simulink model "Rocket_Simulation"  (R2024a)
settings: Solver=VariableStepAuto  StartTime=0.0  StopTime=25  RelTol=1e-3
values from neighbouring files (symbols this model uses):
  g = -9.80665    [OpenRocketDataLoader.m]
undefined symbols (not defined in the file or in its folder): magnitude
libraries: simulink x6, aerolibactuator x1, aerolibatmos2 x1
settings Model: Creator=bennettbabu  LastModifiedBy=mason

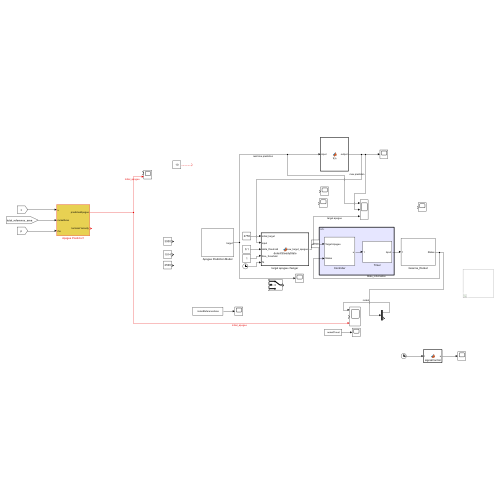
[thumbnail: Simulink's stored preview of the top-level diagram]
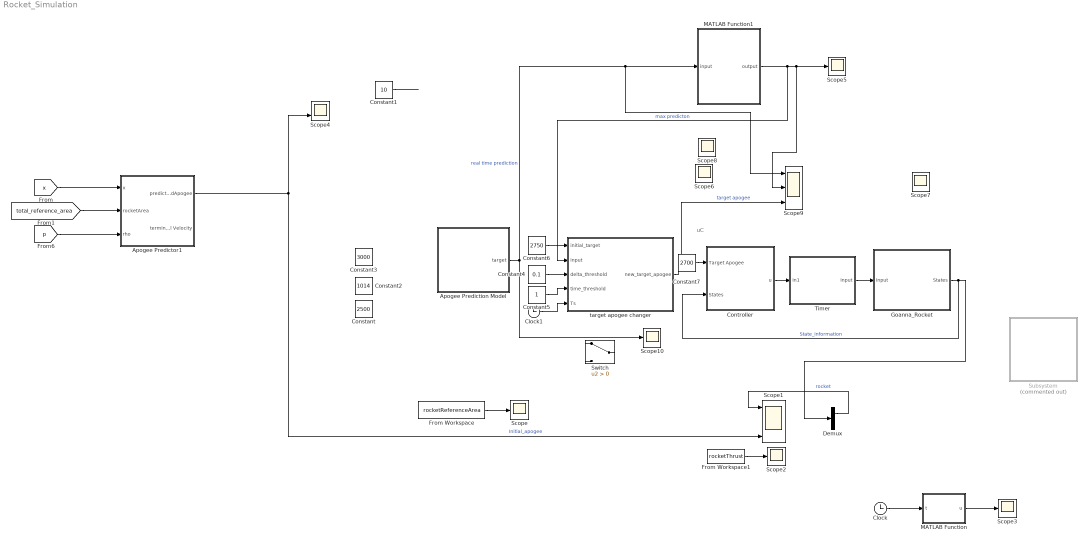
== system Rocket_Simulation ==
  note: uC
  Apogee Prediction Model : Subsystem
  Apogee Predictor1 : Subsystem
  Clock : Clock
  Clock1 : Clock
  Constant : Constant  Value=2500
  Constant1 : Constant  Value=10
  Constant2 : Constant  Value=1014
  Constant3 : Constant  Value=3000
  Constant4 : Constant  Value=0.1
  Constant5 : Constant
  Constant6 : Constant  Value=2750
  Constant7 : Constant  Value=2700
  Controller : Subsystem
  Demux : Demux  Outputs=2
  From Workspace : FromWorkspace  VariableName=rocketReferenceArea
  From Workspace1 : FromWorkspace  VariableName=rocketThrust
  Goanna_Rocket : Subsystem
  MATLAB Function : MATLAB Function  TreatAsAtomicUnit=on
  MATLAB Function1 : MATLAB Function  TreatAsAtomicUnit=on  SystemSampleTime=0.01
  Scope{,2..3,5..8,10} (8 alike) : Scope
  Scope1 : Scope  NumInputPorts=3
  Scope4 : Scope  NumInputPorts=2
  Scope9 : Scope  NumInputPorts=3
  Subsystem : Subsystem  Commented=on
  Switch : Switch  Criteria=u2 > Threshold  SaturateOnIntegerOverflow=off  InputSameDT=off
  Timer : Subsystem
  target apogee changer : MATLAB Function  TreatAsAtomicUnit=on  SystemSampleTime=0.01
  wires:
  Goanna_Rocket/1(States) -> Demux/1, Controller/2(States)  "State_information"
  Controller/1(u) -> Timer/1(In1)
  From Workspace/1 -> Scope/1
  Demux/1 -> Scope1/1  "rocket"
  From Workspace1/1 -> Scope2/1
  Clock/1 -> MATLAB Function/1(t)
  MATLAB Function/1(u) -> Scope3/1
  [p] -> Apogee Predictor1/3(rho)
  [total_reference_area] -> Apogee Predictor1/2(rocketArea)
  [x] -> Apogee Predictor1/1(x)
  MATLAB Function1/1(output) -> target apogee changer/2(input), Scope9/2, Scope5/1  "max predicton"
  Apogee Predictor1/1(predictedApogee) -> Scope1/3, Scope4/2  "Initial_apogee"
  Constant1/1 -> ?
  target apogee changer/1(new_target_apogee) -> Scope9/3  "target apogee"
  Constant4/1 -> target apogee changer/3(delta_threshold)
  Constant5/1 -> target apogee changer/4(time_threshold)
  Clock1/1 -> target apogee changer/5(Ts)
  Apogee Prediction Model/1(target) -> Scope9/1, MATLAB Function1/1(input), Scope10/1  "real time prediction"
  Constant6/1 -> target apogee changer/1(initial_target)
  Constant7/1 -> Controller/1(Target Apogee)
  Timer/1(Input) -> Goanna_Rocket/1(Input)

== system Rocket_Simulation/Apogee Prediction Model ==
  Idealised Curve (Covers the middle Cd and Airbrake Area) : Subsystem
  Multiply : Gain  Gain=1.0
  Scope : Scope
  Terminator : Terminator
  target : Outport
  wires:
  [p] -> Idealised Curve (Covers the middle Cd and Airbrake Area)/2(rho)
  [x] -> Idealised Curve (Covers the middle Cd and Airbrake Area)/1(x)
  Idealised Curve (Covers the middle Cd and Airbrake Area)/1(predictedApogee) -> Multiply/1  "Initial_apogee"
  Multiply/1 -> Scope/1, target/1  "target"
  Idealised Curve (Covers the middle Cd and Airbrake Area)/2(terminal Velocity) -> Terminator/1

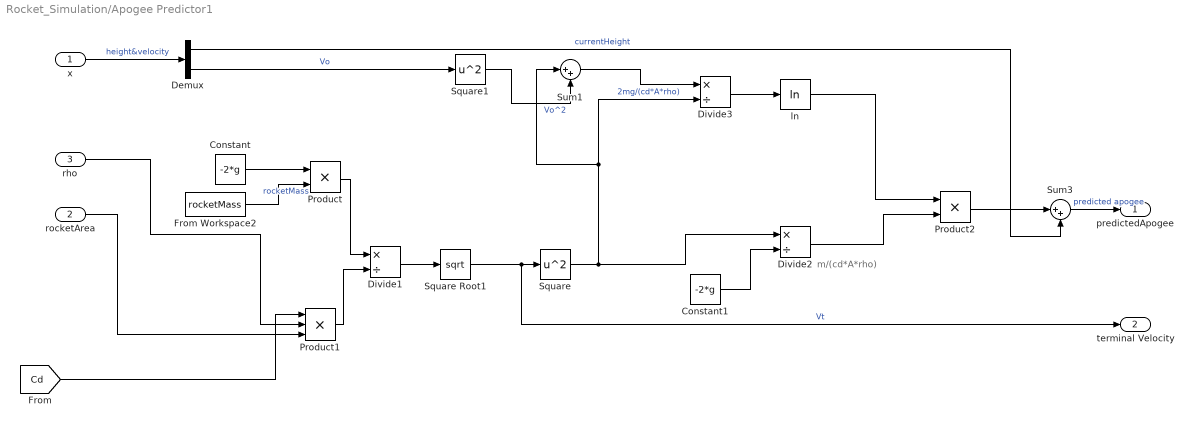
== system Rocket_Simulation/Apogee Predictor1 ==
  note: m/(cd*A*rho)
  x : Inport
  rocketArea : Inport  Port=2
  rho : Inport  Port=3
  Constant : Constant  Value=-2*g
  Constant1 : Constant  Value=-2*g
  Demux : Demux  Outputs=2
  Divide1 : Product  Inputs=*/
  Divide2 : Product  Inputs=*/
  Divide3 : Product  Inputs=*/
  From Workspace2 : FromWorkspace  VariableName=rocketMass
  Product : Product
  Product1 : Product  Inputs=3
  Product2 : Product
  Square : Math  Operator=square
  Square Root1 : Sqrt
  Square1 : Math  Operator=square
  Sum1 : Sum  Inputs=|++
  Sum3 : Sum  Inputs=|++
  ln : Math  Operator=log
  predictedApogee : Outport
  terminal Velocity : Outport  Port=2
  wires:
  Constant/1 -> Product/1
  Product/1 -> Divide1/1
  Product1/1 -> Divide1/2
  [Cd] -> Product1/1
  rho/1 -> Product1/2
  rocketArea/1 -> Product1/3
  Divide1/1 -> Square Root1/1
  Square Root1/1 -> terminal Velocity/1, Square/1  "Vt"
  Product2/1 -> Sum3/1
  ln/1 -> Product2/1
  Divide2/1 -> Product2/2
  Square/1 -> Divide3/2, Sum1/1, Divide2/1  "2mg/(cd*A*rho)"
  Constant1/1 -> Divide2/2
  Divide3/1 -> ln/1
  Square1/1 -> Sum1/2  "Vo^2"
  Sum1/1 -> Divide3/1
  x/1 -> Demux/1  "height&velocity"
  From Workspace2/1 -> Product/2  "rocketMass"
  Demux/2 -> Square1/1  "Vo"
  Demux/1 -> Sum3/2  "currentHeight"
  Sum3/1 -> predictedApogee/1  "predicted apogee"

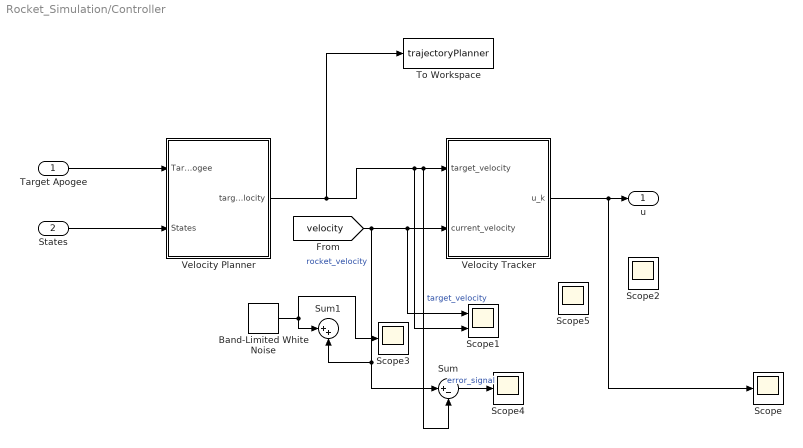
== system Rocket_Simulation/Controller ==
  Target Apogee : Inport
  States : Inport  Port=2
  Band-Limited White Noise : simulink/Sources/Band-Limited White Noise  Cov=[0.00001]  Ts=0.001  seed=[23341]
  Scope{,2..5} (5 alike) : Scope
  Scope1 : Scope  NumInputPorts=2
  Sum : Sum  Inputs=|+-
  Sum1 : Sum  Inputs=|++
  To Workspace : ToWorkspace  VariableName=trajectoryPlanner  SaveFormat=Timeseries  SampleTime=-1
  Velocity Planner : Subsystem
  Velocity Tracker : Subsystem
  u : Outport
  wires:
  Target Apogee/1 -> Velocity Planner/1(Target Apogee)
  States/1 -> Velocity Planner/2(States)
  Velocity Tracker/1(u_k) -> Scope/1, u/1
  [velocity] -> Sum1/2, Sum/1, Velocity Tracker/2(current_velocity), Scope1/1  "rocket_velocity"
  Velocity Planner/1(target_velocity) -> To Workspace/1, Sum/2, Velocity Tracker/1(target_velocity), Scope1/2  "target_velocity"
  Band-Limited White Noise/1 -> Scope3/1, Sum1/1
  Sum/1 -> Scope4/1  "error_signal"

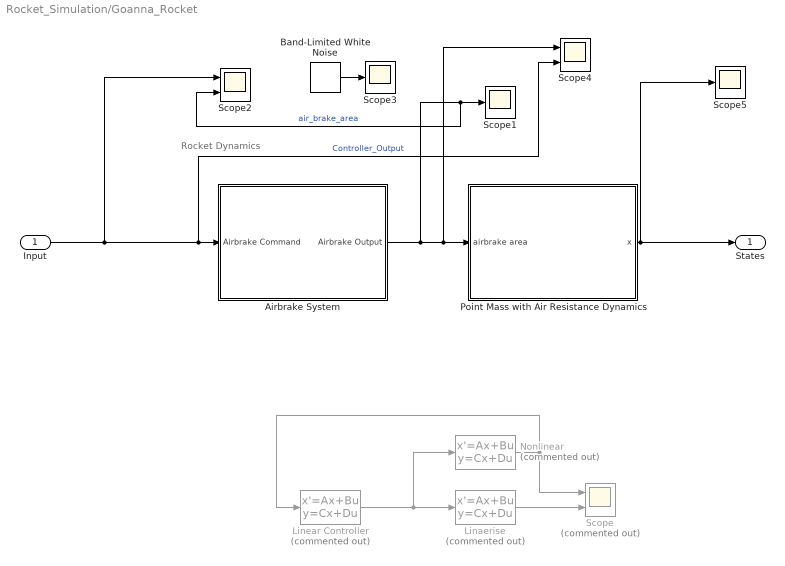
== system Rocket_Simulation/Goanna_Rocket ==
  note: Rocket Dynamics
  Input : Inport
  Airbrake System : Subsystem
      mask Display: image('airbrake.png');
  Band-Limited White Noise : simulink/Sources/Band-Limited White Noise  Cov=[0.0001]  Ts=0.1  seed=[23341]
  "Linaerise " : StateSpace  Commented=on  InitialCondition=0
  Linear Controller : StateSpace  Commented=on  InitialCondition=0
  Nonlinear : StateSpace  Commented=on  InitialCondition=0
  "Point Mass with Air Resistance Dynamics " : Subsystem
      mask Display: image('rocket.jpeg');
  Scope : Scope  Commented=on  NumInputPorts=2
  Scope1 : Scope
  Scope2 : Scope  NumInputPorts=2
  Scope3 : Scope
  Scope4 : Scope  NumInputPorts=2
  Scope5 : Scope
  States : Outport
  wires:
  Linear Controller/1 -> Nonlinear/1, "Linaerise "/1
  Nonlinear/1 -> Linear Controller/1, Scope/1
  "Linaerise "/1 -> Scope/2
  Input/1 -> Scope2/1, Scope4/2, Airbrake System/1(Airbrake Command)  "Controller_Output"
  Airbrake System/1(Airbrake Output) -> Scope4/1, "Point Mass with Air Resistance Dynamics "/1(airbrake area), Scope2/2, Scope1/1  "air_brake_area"
  Band-Limited White Noise/1 -> Scope3/1
  "Point Mass with Air Resistance Dynamics "/1(x) -> Scope5/1, States/1

== system Rocket_Simulation/Subsystem ==
  wires:
  ? -> ?

== system Rocket_Simulation/Timer ==
  In1 : Inport
  Clock : Clock
  Constant1 : Constant  Value=0
  Switch : Switch  Criteria=u2 > Threshold  Threshold=3  SaturateOnIntegerOverflow=off  InputSameDT=off
  Input : Outport
  wires:
  Switch/1 -> Input/1
  Clock/1 -> Switch/2
  In1/1 -> Switch/1
  Constant1/1 -> Switch/3

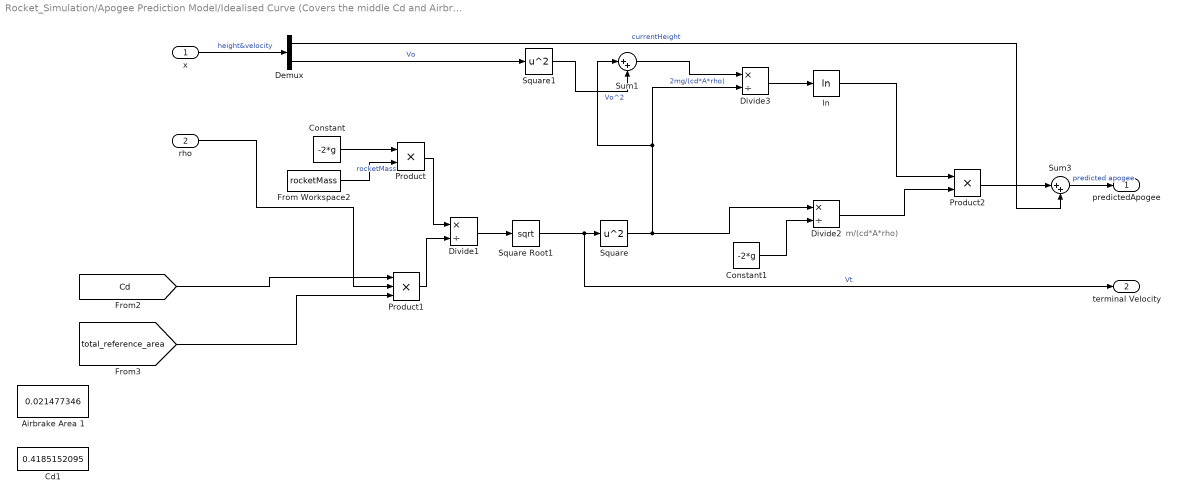
== system Rocket_Simulation/Apogee Prediction Model/Idealised Curve (Covers the middle Cd and Airbrake Area) ==
  note: m/(cd*A*rho)
  x : Inport
  rho : Inport  Port=2
  Airbrake Area 1 : Constant  Value=0.021477346
  Cd1 : Constant  Value=0.4185152095
  Constant : Constant  Value=-2*g
  Constant1 : Constant  Value=-2*g
  Demux : Demux  Outputs=2
  Divide1 : Product  Inputs=*/
  Divide2 : Product  Inputs=*/
  Divide3 : Product  Inputs=*/
  From Workspace2 : FromWorkspace  VariableName=rocketMass
  Product : Product
  Product1 : Product  Inputs=3
  Product2 : Product
  Square : Math  Operator=square
  Square Root1 : Sqrt
  Square1 : Math  Operator=square
  Sum1 : Sum  Inputs=|++
  Sum3 : Sum  Inputs=|++
  ln : Math  Operator=log
  predictedApogee : Outport
  terminal Velocity : Outport  Port=2
  wires:
  Constant/1 -> Product/1
  Product/1 -> Divide1/1
  Product1/1 -> Divide1/2
  [Cd] -> Product1/1
  rho/1 -> Product1/2
  [total_reference_area] -> Product1/3
  Divide1/1 -> Square Root1/1
  Square Root1/1 -> terminal Velocity/1, Square/1  "Vt"
  Product2/1 -> Sum3/1
  ln/1 -> Product2/1
  Divide2/1 -> Product2/2
  Square/1 -> Divide3/2, Sum1/1, Divide2/1  "2mg/(cd*A*rho)"
  Constant1/1 -> Divide2/2
  Divide3/1 -> ln/1
  Square1/1 -> Sum1/2  "Vo^2"
  Sum1/1 -> Divide3/1
  x/1 -> Demux/1  "height&velocity"
  From Workspace2/1 -> Product/2  "rocketMass"
  Demux/2 -> Square1/1  "Vo"
  Demux/1 -> Sum3/2  "currentHeight"
  Sum3/1 -> predictedApogee/1  "predicted apogee"

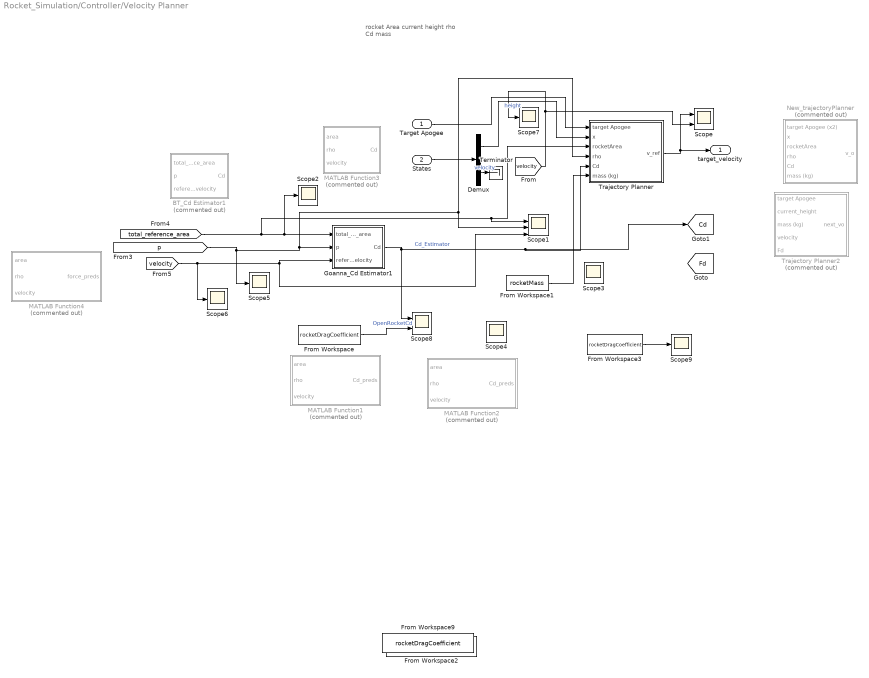
== system Rocket_Simulation/Controller/Velocity Planner ==
  note: rocket Area
      | current height
      | rho
      | Cd
      | mass
  Target Apogee : Inport
  States : Inport  Port=2
  BT_Cd Estimator1 : Subsystem  Commented=on
  Demux : Demux  Outputs=2
  From Workspace{,2..3,9} (4 alike) : FromWorkspace  VariableName=rocketDragCoefficient
  From Workspace1 : FromWorkspace  VariableName=rocketMass
  Goanna_Cd Estimator1 : Subsystem
  MATLAB Function1 : MATLAB Function  Commented=on  TreatAsAtomicUnit=on
  MATLAB Function2 : MATLAB Function  Commented=on  TreatAsAtomicUnit=on
  MATLAB Function3 : MATLAB Function  Commented=on  TreatAsAtomicUnit=on
  MATLAB Function4 : MATLAB Function  Commented=on  TreatAsAtomicUnit=on
  New_trajectoryPlanner : Subsystem  Commented=on
  Scope : Scope  NumInputPorts=2
  Scope1 : Scope  NumInputPorts=4
  Scope{2..7,9} (7 alike) : Scope
  Scope8 : Scope  NumInputPorts=2
  Terminator : Terminator
  Trajectory Planner : Subsystem
  Trajectory Planner2 : Subsystem  Commented=on
  target_velocity : Outport
  tag scope: Cd=global, Fd=global
  wires:
  States/1 -> Demux/1
  Demux/1 -> Trajectory Planner/2(x)  "height"
  Target Apogee/1 -> Trajectory Planner/1(target Apogee)
  [total_reference_area] -> Trajectory Planner/3(rocketArea), Scope1/2, Goanna_Cd Estimator1/1(total_reference_area), Scope2/1
  Trajectory Planner/1(v_ref) -> Scope/1, target_velocity/1
  [velocity] -> Goanna_Cd Estimator1/3(reference_velocity), Scope1/4, Scope6/1
  [velocity] -> Scope/2, Scope7/1
  Goanna_Cd Estimator1/1(Cd) -> Scope8/1, Trajectory Planner/5(Cd), [Cd]  "Cd_Estimator"
  From Workspace1/1 -> Trajectory Planner/6(mass (kg))
  [p] -> Goanna_Cd Estimator1/2(p), Trajectory Planner/4(rho), Scope1/3, Scope5/1
  Demux/2 -> Terminator/1  "velocity"
  From Workspace/1 -> Scope8/2  "OpenRocketCd"
  From Workspace3/1 -> Scope9/1

== system Rocket_Simulation/Controller/Velocity Tracker ==
  target_velocity : Inport
  current_velocity : Inport  Port=2
  MATLAB Function2 : MATLAB Function  Commented=on  TreatAsAtomicUnit=on
  MATLAB Function3 : MATLAB Function  TreatAsAtomicUnit=on
  Scope : Scope
  Scope2 : Scope
  u_k : Outport
  wires:
  MATLAB Function3/1(u_k) -> Scope/1, u_k/1  "switched model"
  target_velocity/1 -> MATLAB Function3/1(Vref)
  current_velocity/1 -> MATLAB Function3/2(x)

== system Rocket_Simulation/Goanna_Rocket/Airbrake System ==
  Airbrake Command : Inport
  Nonlinear Second-Order Actuator : aerolibactuator/Nonlinear Second-Order Actuator  wn_fin=5  z_fin=0.7  fin_max=maxAirbrakeArea_Goanna  fin_min=0  fin_maxrate=315*pi/180  fin_act_0=0  fin_act_vel=0
  Scope : Scope  NumInputPorts=2
  Scope1 : Scope
  Square Wave Generator : SignalGenerator  Commented=on  WaveForm=square  Amplitude=0.01  Units=rad/sec
  Airbrake Output : Outport
  wires:
  Nonlinear Second-Order Actuator/1 -> Scope1/1, Scope/2, Airbrake Output/1
  Airbrake Command/1 -> Nonlinear Second-Order Actuator/1, Scope/1

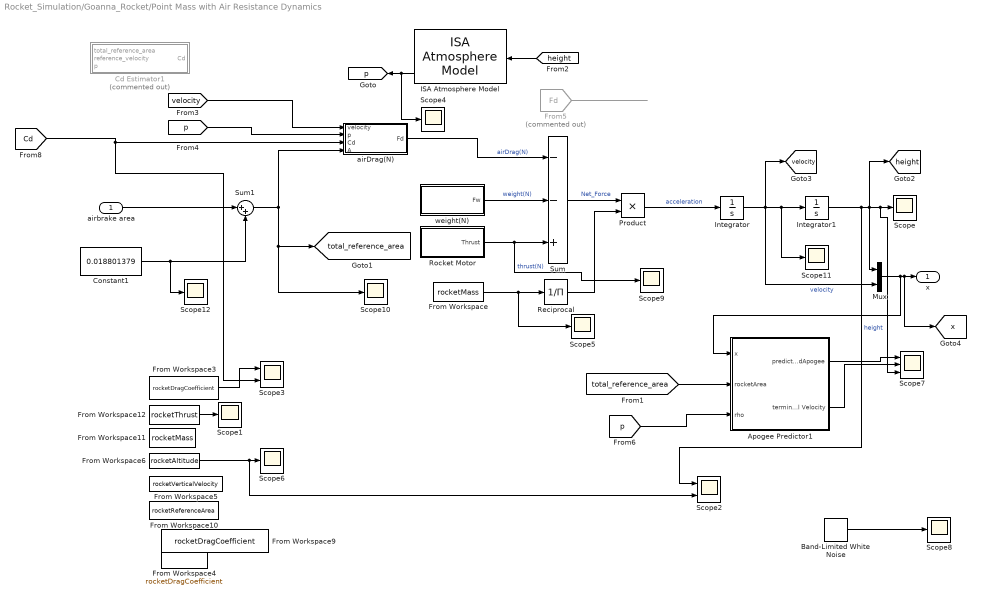
== system Rocket_Simulation/Goanna_Rocket/Point Mass with Air Resistance Dynamics  ==
  airbrake area : Inport
  Apogee Predictor1 : Subsystem
  Band-Limited White Noise : simulink/Sources/Band-Limited White Noise  Cov=[0.1]  Ts=0.1  seed=[23341]
  Cd Estimator1 : Subsystem  Commented=on
  Constant1 : Constant  Value=0.018801379
  From Workspace : FromWorkspace  VariableName=rocketMass
  From Workspace10 : FromWorkspace  VariableName=rocketReferenceArea
  From Workspace11 : FromWorkspace  VariableName=rocketMass
  From Workspace12 : FromWorkspace  VariableName=rocketThrust
  From Workspace3 : FromWorkspace  VariableName=rocketDragCoefficient
  From Workspace4 : FromWorkspace  VariableName=rocketDragCoefficient
  From Workspace5 : FromWorkspace  VariableName=rocketVerticalVelocity
  From Workspace6 : FromWorkspace  VariableName=rocketAltitude
  From Workspace9 : FromWorkspace  VariableName=rocketDragCoefficient
  From5 : From  Commented=on  GotoTag=Fd  TagVisibility=global
  ISA Atmosphere Model : aerolibatmos2/ISA Atmosphere Model  useExtended=off  action=Warning  custom=on  viscosityOut=off  g=9.80665  gamma=1.4  R=287.0531  L=0.0065  h_trop=11000  h_strat=20000  rho0=1.225  P0=101325  T0=288.15  h0=0  S=110.4  Tref=273.15  muref=1.716e-5
  Integrator : Integrator
  Integrator1 : Integrator
  Mux : Mux  Inputs=2
  Product : Product
  Reciprocal : Product  Inputs=/
  "Rocket Motor " : Subsystem
  Scope{,1,4..6,8..12} (10 alike) : Scope
  Scope2 : Scope  NumInputPorts=2
  Scope3 : Scope  NumInputPorts=2
  Scope7 : Scope  NumInputPorts=3
  Sum : Sum  Inputs=--+
  Sum1 : Sum  Inputs=|++
  airDrag(N) : Subsystem
  weight(N) : Subsystem
  x : Outport
  tag scope: height=global, p=global, total_reference_area=global, velocity=global, x=global
  wires:
  "Rocket Motor "/1(Thrust) -> Scope9/1, Sum/3  "thrust(N)"
  weight(N)/1(Fw) -> Sum/2  "weight(N)"
  Sum/1 -> Product/1  "Net_Force"
  ISA Atmosphere Model/4 -> Scope4/1, [p]
  [height] -> ISA Atmosphere Model/1
  [velocity] -> airDrag(N)/1(velocity)
  [p] -> airDrag(N)/2(p)
  Product/1 -> Integrator/1  "acceleration"
  Integrator/1 -> [velocity], Scope11/1, Integrator1/1, Mux/2  "velocity"
  Integrator1/1 -> Scope2/1, Mux/1, [height], Scope7/3, Scope/1  "height"
  Mux/1 -> Apogee Predictor1/1(x), [x], x/1
  Reciprocal/1 -> Product/2
  From Workspace/1 -> Scope5/1, Reciprocal/1
  From Workspace12/1 -> Scope1/1
  airbrake area/1 -> Sum1/1
  Sum1/1 -> Scope10/1, [total_reference_area], airDrag(N)/4(A)
  Constant1/1 -> Scope12/1, Sum1/2
  [Cd] -> Scope3/2, airDrag(N)/3(Cd)
  From Workspace3/1 -> Scope3/1
  From5/1 -> ?
  airDrag(N)/1(Fd) -> Sum/1  "airDrag(N)"
  From Workspace6/1 -> Scope2/2, Scope6/1
  [total_reference_area] -> Apogee Predictor1/2(rocketArea)
  [p] -> Apogee Predictor1/3(rho)
  Apogee Predictor1/1(predictedApogee) -> Scope7/1
  Apogee Predictor1/2(terminal Velocity) -> Scope7/2
  Band-Limited White Noise/1 -> Scope8/1

== system Rocket_Simulation/Controller/Velocity Planner/BT_Cd Estimator1 ==
  total_reference_area : Inport
  p : Inport  Port=2
  reference_velocity : Inport  Port=3
  Gain : Gain  Gain=0.92
  Rocket Specific Cd Estimator : MATLAB Function  TreatAsAtomicUnit=on
  Cd : Outport
  wires:
  Rocket Specific Cd Estimator/1(Cd) -> Gain/1
  total_reference_area/1 -> Rocket Specific Cd Estimator/1(SA)
  reference_velocity/1 -> Rocket Specific Cd Estimator/2(V)
  p/1 -> Rocket Specific Cd Estimator/3(rho)
  Gain/1 -> Cd/1

== system Rocket_Simulation/Controller/Velocity Planner/Goanna_Cd Estimator1 ==
  total_reference_area : Inport
  p : Inport  Port=2
  reference_velocity : Inport  Port=3
  Gain : Gain  Gain=1.18
  Rocket Specific Cd Estimator : MATLAB Function  TreatAsAtomicUnit=on
  Scope : Scope
  Cd : Outport
  wires:
  Rocket Specific Cd Estimator/1(Cd) -> Gain/1
  total_reference_area/1 -> Scope/1, Rocket Specific Cd Estimator/1(area)
  reference_velocity/1 -> Rocket Specific Cd Estimator/3(velocity)
  p/1 -> Rocket Specific Cd Estimator/2(rho)
  Gain/1 -> Cd/1

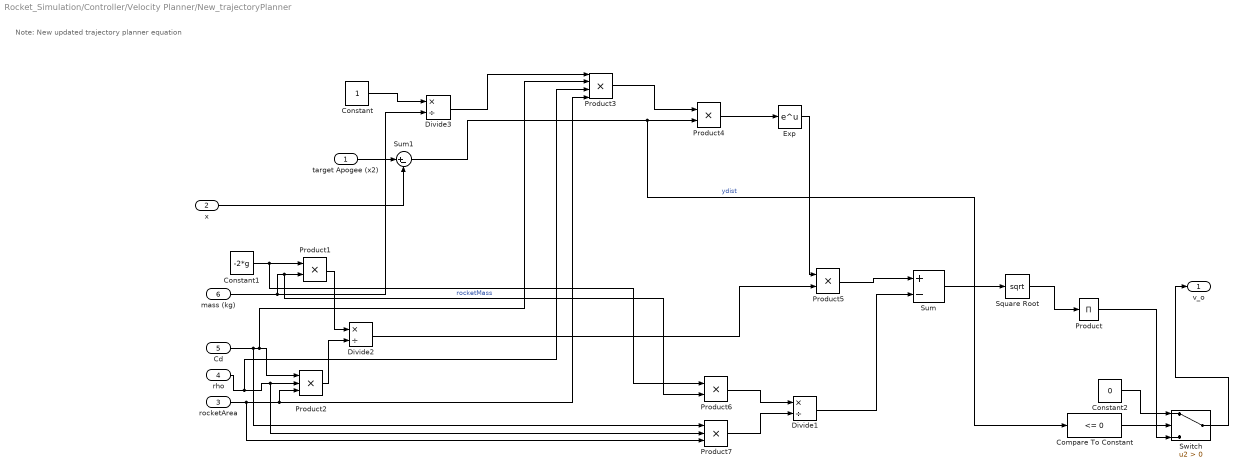
== system Rocket_Simulation/Controller/Velocity Planner/New_trajectoryPlanner ==
  note: Note: New updated trajectory planner equation
  target Apogee (x2) : Inport
  x : Inport  Port=2
  rocketArea : Inport  Port=3
  rho : Inport  Port=4
  Cd : Inport  Port=5
  mass (kg) : Inport  Port=6
  Compare To Constant : simulink/Logic and Bit Operations/Compare To Constant  relop=<=  const=0  OutDataTypeStr=boolean
  Constant : Constant
  Constant1 : Constant  Value=-2*g
  Constant2 : Constant  Value=0
  Divide1 : Product  Inputs=*/
  Divide2 : Product  Inputs=*/
  Divide3 : Product  Inputs=*/
  Exp : Math
  Product : Product  Inputs=1
  Product{1,4..6} (4 alike) : Product
  Product2 : Product  Inputs=3
  Product3 : Product  Inputs=4
  Product7 : Product  Inputs=3
  Square Root : Sqrt
  Sum : Sum  Inputs=+-
  Sum1 : Sum  Inputs=|+-
  Switch : Switch  Criteria=u2 > Threshold  SaturateOnIntegerOverflow=off  InputSameDT=off
  v_o : Outport
  wires:
  target Apogee (x2)/1 -> Sum1/1
  Product2/1 -> Divide2/2
  Cd/1 -> Product7/1, Product3/2, Product2/1
  rocketArea/1 -> Product7/3, Product3/4, Product2/3
  Product1/1 -> Divide2/1
  Constant1/1 -> Product6/1, Product1/1
  rho/1 -> Product3/3, Product7/2, Product2/2
  mass (kg)/1 -> Divide3/2, Product6/2, Product1/2  "rocketMass"
  Divide3/1 -> Product3/1
  Product3/1 -> Product4/1
  Product4/1 -> Exp/1
  Divide2/1 -> Product5/2
  Exp/1 -> Product5/1
  Product5/1 -> Sum/1
  Divide1/1 -> Sum/2
  Product6/1 -> Divide1/1
  Product7/1 -> Divide1/2
  Sum/1 -> Square Root/1
  Constant/1 -> Divide3/1
  Switch/1 -> v_o/1
  Compare To Constant/1 -> Switch/2
  Sum1/1 -> Compare To Constant/1, Product4/2  "ydist"
  Constant2/1 -> Switch/1
  Square Root/1 -> Product/1
  Product/1 -> Switch/3
  x/1 -> Sum1/2

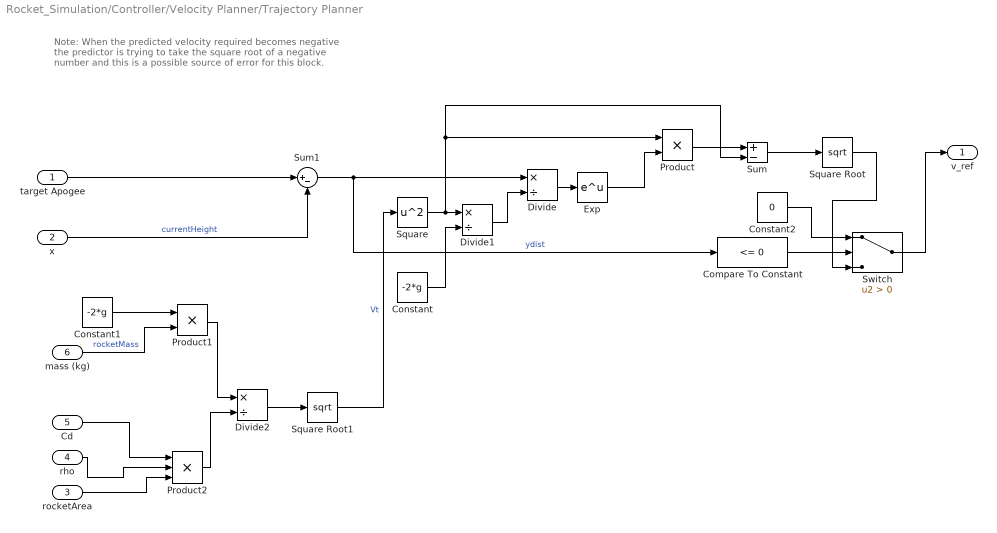
== system Rocket_Simulation/Controller/Velocity Planner/Trajectory Planner ==
  note: Note: When the predicted velocity required becomes negative the predictor is trying to take the square root of a negative number and this is a possible source of error for this block.
  target Apogee : Inport
  x : Inport  Port=2
  rocketArea : Inport  Port=3
  rho : Inport  Port=4
  Cd : Inport  Port=5
  mass (kg) : Inport  Port=6
  Compare To Constant : simulink/Logic and Bit Operations/Compare To Constant  relop=<=  const=0  OutDataTypeStr=boolean
  Constant : Constant  Value=-2*g
  Constant1 : Constant  Value=-2*g
  Constant2 : Constant  Value=0
  Divide : Product  Inputs=*/
  Divide1 : Product  Inputs=*/
  Divide2 : Product  Inputs=*/
  Exp : Math
  Product : Product
  Product1 : Product
  Product2 : Product  Inputs=3
  Square : Math  Operator=square
  Square Root : Sqrt
  Square Root1 : Sqrt
  Sum : Sum  Inputs=+-
  Sum1 : Sum  Inputs=|+-
  Switch : Switch  Criteria=u2 > Threshold  SaturateOnIntegerOverflow=off  InputSameDT=off
  v_ref : Outport
  wires:
  Sum/1 -> Square Root/1
  Product/1 -> Sum/1
  Exp/1 -> Product/2
  Divide/1 -> Exp/1
  Sum1/1 -> Compare To Constant/1, Divide/1  "ydist"
  Constant/1 -> Divide1/2
  Divide1/1 -> Divide/2
  Square/1 -> Sum/2, Product/1, Divide1/1
  target Apogee/1 -> Sum1/1
  Product2/1 -> Divide2/2
  Square Root1/1 -> Square/1  "Vt"
  Cd/1 -> Product2/1
  Divide2/1 -> Square Root1/1
  rocketArea/1 -> Product2/3
  Product1/1 -> Divide2/1
  Constant1/1 -> Product1/1
  rho/1 -> Product2/2
  mass (kg)/1 -> Product1/2  "rocketMass"
  x/1 -> Sum1/2  "currentHeight"
  Compare To Constant/1 -> Switch/2
  Constant2/1 -> Switch/1
  Square Root/1 -> Switch/3
  Switch/1 -> v_ref/1

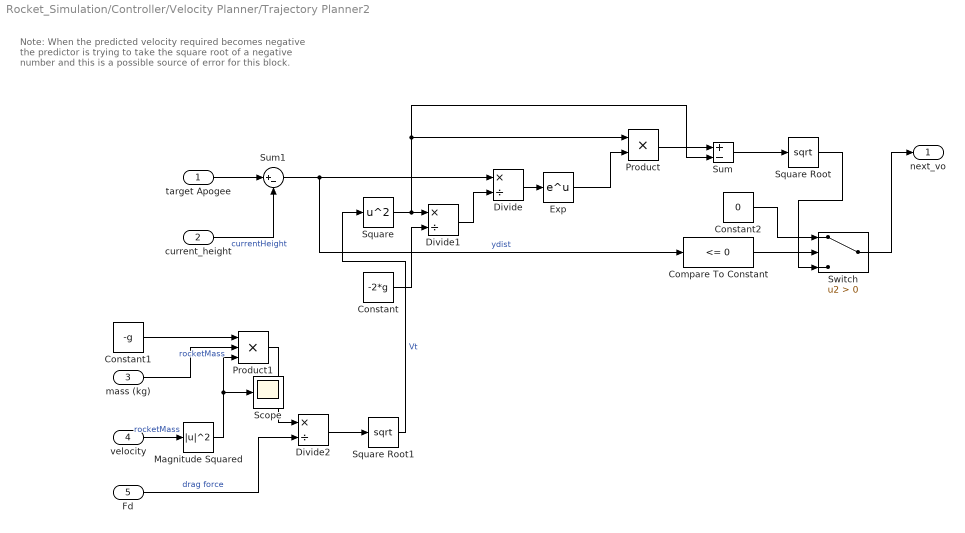
== system Rocket_Simulation/Controller/Velocity Planner/Trajectory Planner2 ==
  note: Note: When the predicted velocity required becomes negative the predictor is trying to take the square root of a negative number and this is a possible source of error for this block.
  target Apogee : Inport
  current_height : Inport  Port=2
  mass (kg) : Inport  Port=3
  velocity : Inport  Port=4
  Fd : Inport  Port=5
  Compare To Constant : simulink/Logic and Bit Operations/Compare To Constant  relop=<=  const=0  OutDataTypeStr=boolean
  Constant : Constant  Value=-2*g
  Constant1 : Constant  Value=-g
  Constant2 : Constant  Value=0
  Divide : Product  Inputs=*/
  Divide1 : Product  Inputs=*/
  Divide2 : Product  Inputs=*/
  Exp : Math
  Magnitude Squared : Math  Operator=magnitude^2
  Product : Product
  Product1 : Product  Inputs=3
  Scope : Scope
  Square : Math  Operator=square
  Square Root : Sqrt
  Square Root1 : Sqrt
  Sum : Sum  Inputs=+-
  Sum1 : Sum  Inputs=|+-
  Switch : Switch  Criteria=u2 > Threshold  SaturateOnIntegerOverflow=off  InputSameDT=off
  next_vo : Outport
  wires:
  Sum/1 -> Square Root/1
  Product/1 -> Sum/1
  Exp/1 -> Product/2
  Divide/1 -> Exp/1
  Sum1/1 -> Compare To Constant/1, Divide/1  "ydist"
  Constant/1 -> Divide1/2
  Divide1/1 -> Divide/2
  Square/1 -> Sum/2, Product/1, Divide1/1
  target Apogee/1 -> Sum1/1
  Square Root1/1 -> Square/1  "Vt"
  Divide2/1 -> Square Root1/1
  Product1/1 -> Divide2/1
  Constant1/1 -> Product1/1
  mass (kg)/1 -> Product1/2  "rocketMass"
  current_height/1 -> Sum1/2  "currentHeight"
  Compare To Constant/1 -> Switch/2
  Constant2/1 -> Switch/1
  Square Root/1 -> Switch/3
  Switch/1 -> next_vo/1
  Fd/1 -> Divide2/2  "drag force"
  velocity/1 -> Magnitude Squared/1  "rocketMass"
  Magnitude Squared/1 -> Product1/3, Scope/1

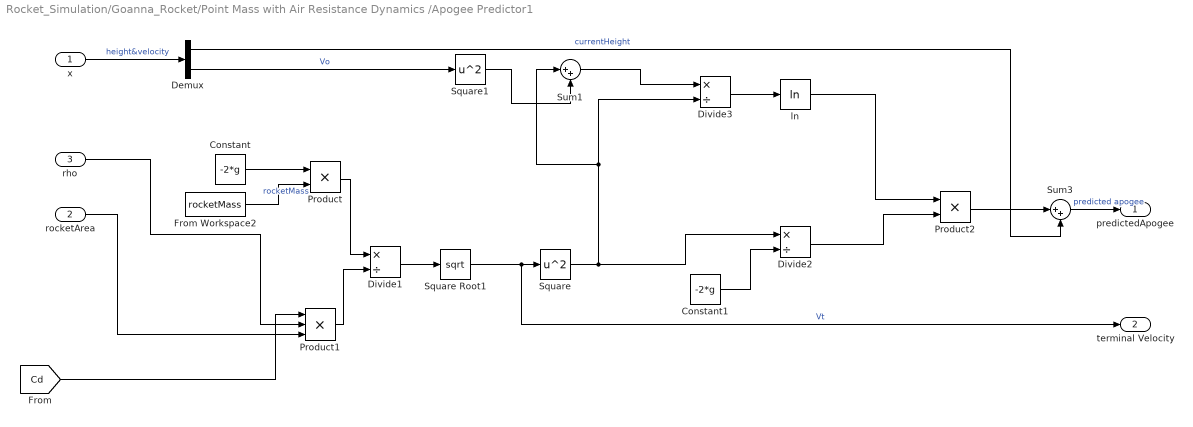
== system Rocket_Simulation/Goanna_Rocket/Point Mass with Air Resistance Dynamics /Apogee Predictor1 ==
  x : Inport
  rocketArea : Inport  Port=2
  rho : Inport  Port=3
  Constant : Constant  Value=-2*g
  Constant1 : Constant  Value=-2*g
  Demux : Demux  Outputs=2
  Divide1 : Product  Inputs=*/
  Divide2 : Product  Inputs=*/
  Divide3 : Product  Inputs=*/
  From Workspace2 : FromWorkspace  VariableName=rocketMass
  Product : Product
  Product1 : Product  Inputs=3
  Product2 : Product
  Square : Math  Operator=square
  Square Root1 : Sqrt
  Square1 : Math  Operator=square
  Sum1 : Sum  Inputs=|++
  Sum3 : Sum  Inputs=|++
  ln : Math  Operator=log
  predictedApogee : Outport
  terminal Velocity : Outport  Port=2
  wires:
  Constant/1 -> Product/1
  Product/1 -> Divide1/1
  Product1/1 -> Divide1/2
  [Cd] -> Product1/1
  rho/1 -> Product1/2
  rocketArea/1 -> Product1/3
  Divide1/1 -> Square Root1/1
  Square Root1/1 -> terminal Velocity/1, Square/1  "Vt"
  Product2/1 -> Sum3/1
  ln/1 -> Product2/1
  Divide2/1 -> Product2/2
  Square/1 -> Divide3/2, Sum1/1, Divide2/1
  Constant1/1 -> Divide2/2
  Divide3/1 -> ln/1
  Square1/1 -> Sum1/2
  Sum1/1 -> Divide3/1
  x/1 -> Demux/1  "height&velocity"
  From Workspace2/1 -> Product/2  "rocketMass"
  Demux/2 -> Square1/1  "Vo"
  Demux/1 -> Sum3/2  "currentHeight"
  Sum3/1 -> predictedApogee/1  "predicted apogee"

== system Rocket_Simulation/Goanna_Rocket/Point Mass with Air Resistance Dynamics /Cd Estimator1 ==
  total_reference_area : Inport
  reference_velocity : Inport  Port=2
  p : Inport  Port=3
  Rocket Specific Cd Estimator : MATLAB Function  TreatAsAtomicUnit=on
  Cd : Outport
  wires:
  Rocket Specific Cd Estimator/1(Cd) -> Cd/1
  total_reference_area/1 -> Rocket Specific Cd Estimator/1(SA)
  reference_velocity/1 -> Rocket Specific Cd Estimator/2(V)
  p/1 -> Rocket Specific Cd Estimator/3(rho)

== system Rocket_Simulation/Goanna_Rocket/Point Mass with Air Resistance Dynamics /Rocket Motor  ==
  From Workspace12 : FromWorkspace  VariableName=rocketThrust
  Gain : Gain  Gain=1.0
  Thrust : Outport
  wires:
  From Workspace12/1 -> Gain/1
  Gain/1 -> Thrust/1

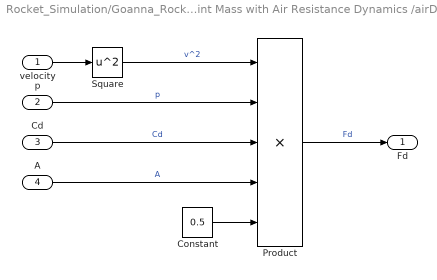
== system Rocket_Simulation/Goanna_Rocket/Point Mass with Air Resistance Dynamics /airDrag(N) ==
  velocity : Inport
  p : Inport  Port=2
  Cd : Inport  Port=3
  A : Inport  Port=4
  Constant : Constant  Value=0.5
  Product : Product  Inputs=5
  Square : Math  Operator=square
  Fd : Outport
  wires:
  velocity/1 -> Square/1
  Square/1 -> Product/1  "v^2"
  p/1 -> Product/2  "p"
  Cd/1 -> Product/3  "Cd"
  A/1 -> Product/4  "A"
  Constant/1 -> Product/5
  Product/1 -> Fd/1  "Fd"

== system Rocket_Simulation/Goanna_Rocket/Point Mass with Air Resistance Dynamics /weight(N) ==
  From Workspace11 : FromWorkspace  VariableName=rocketMass
  gravity : Gain  Gain=9.80665
  Fw : Outport
  wires:
  From Workspace11/1 -> gravity/1
  gravity/1 -> Fw/1

== matlab function Rocket_Simulation/Controller/Velocity Planner/MATLAB Function3 ==
  data: area input; Cd output; rho input; velocity input
function Cd = cd_estimator(area, rho, velocity)
    % coefficients = [intercept, Area, Density, Velocity, Area^2, Area*Density, Area*Velocity, Density^2, Velocity^2];
    coefficients = [1.271359304570330, -89.2957223507969, -0.139915015095874, -0.000642306508177183, 2402.82168908320, 5.06245068661305, 0.0110556725929730, 0.00208924419408200, 6.72989011187282e-07];
    
    % Manually generate polynomial features for scalar inputs
    X_pred_poly = [1, ... % Intercept term
                   area, ... % Area
                   rho, ... % Density
                   velocity, ... % Velocity
                   area^2, ... % Area^2
                   area * rho, ... % Area * Density
                   area * velocity, ... % Area * Velocity
                   rho^2, ... % Density^2
                   velocity^2]; % Velocity^2
    
    Cd = X_pred_poly * coefficients';
end

== matlab function Rocket_Simulation/Controller/Velocity Tracker/MATLAB Function3 ==
  data: Vref input; x input; u_k output
function u_k = fcn(Vref, x)
    %% Measurements

    xref_k = Vref;
    x_k = x; % measured system states
    u_k = 0; % Initialize u_k

    if x <= 40
        K = -0.557604560965188;
    elseif x <= 80
        K = -0.149050395144053;
    elseif x <= 140
        K = -0.050007237207140;
    elseif x <= 180
        K = -0.021944352703524;
    else
        K = -0.035; % Default value for K
    end

    % Calculate control signal
    u_k = -K * (x_k - xref_k);

    % Ensure u_k is non-negative
    if u_k < 0
        u_k = 0;
    end
    
    return
end

== matlab function Rocket_Simulation/MATLAB Function ==
  data: t input; u output; maxAirbrakeArea_Skink parameter
function u = signalControl(t,maxAirbrakeArea_Skink)
    % signalControl function to control the signal 'u'
    % Inputs: t - time from the simulation environment
    % Outputs: u - the signal output
    
    % Initialize u
    u = 0;
    
    % Check the time and set u accordingly
    if t >= 3 && t < 15
        u = maxAirbrakeArea_Skink;
    elseif t >= 15
        u = 0;
    end
end

== matlab function Rocket_Simulation/Controller/Velocity Planner/MATLAB Function1 ==
  data: area input; Cd_preds output; rho input; velocity input
function Cd_preds = predict_drag_coefficients(area, rho, velocity)
    % Load model parameters from the .mat file
    params = load('model_params.mat');
    area
    rho
    velocity = abs(velocity)
    % Generate predictions for a grid of velocities
    force_preds = arrayfun(@(v) poly_predict(area, rho, v, params), velocity);
    
    % Check if any of the inputs are zero
    if area ~= 0 && rho ~= 0 && all(velocity ~= 0)
        % Calculate Cd for each velocity

        Cd_preds = arrayfun(@(f, v) f / (0.5 * rho * area * v^2), force_preds, velocity)
        if Cd_preds <= 0
            Cd_preds = 0.386598;
        end 
    else
        % Assign default value if any input is zero
        Cd_preds = 0.386598;
    end
end

function y_pred = poly_predict(area, rho, velocity, params)
    % Extract the parameters
    scaler_X_mean = params.scaler_X_mean;
    scaler_X_std = params.scaler_X_std;
    scaler_y_mean = params.scaler_y_mean;
    scaler_y_std = params.scaler_y_std;
    coefficients = params.coefficients;
    intercept = params.intercept;

    % Standardize input features (This is required because the GPR was trained this way)
    X = [(area - scaler_X_mean(1)) / scaler_X_std(1), ...
         (rho - scaler_X_mean(2)) / scaler_X_std(2), ...
         (velocity - scaler_X_mean(3)) / scaler_X_std(3)];

    % Compute polynomial features up to the desired degree
    degree = 3;
    X_poly = get_poly_features(X, degree);

    % Predict using the polynomial model
    y_scaled = sum(coefficients .* X_poly) + intercept;

    % Inverse standardization of the prediction
    y_pred = y_scaled * scaler_y_std + scaler_y_mean;
end

function X_poly = get_poly_features(X, degree)
    % Generate polynomial features up to the desired degree
    n = length(X);
    X_poly = 1;  % constant bias term

    for d = 1:degree
        combos = nchoosek(repmat(1:n, 1, d), d);
        combos = unique(sort(combos, 2), 'rows');
        for i = 1:size(combos, 1)
            term = prod(X(combos(i, :)));
            X_poly = [X_poly, term];
        end
    end
end

== matlab function Rocket_Simulation/Controller/Velocity Planner/Goanna_Cd Estimator1/Rocket Specific Cd Estimator ==
  data: area input; rho input; Cd output; velocity input
function Cd = cd_estimator(area, rho, velocity)
    % coefficients = [intercept, Area, Density, Velocity, Area^2, Area*Density, Area*Velocity, Density^2, Velocity^2];
    coefficients = [1.271359304570330, -89.2957223507969, -0.139915015095874, -0.000642306508177183, 2402.82168908320, 5.06245068661305, 0.0110556725929730, 0.00208924419408200, 6.72989011187282e-07];
    
    % Manually generate polynomial features for scalar inputs
    X_pred_poly = [1, ... % Intercept term
                   area, ... % Area
                   rho, ... % Density
                   velocity, ... % Velocity
                   area^2, ... % Area^2
                   area * rho, ... % Area * Density
                   area * velocity, ... % Area * Velocity
                   rho^2, ... % Density^2
                   velocity^2]; % Velocity^2
    
    Cd = X_pred_poly * coefficients';
end

== matlab function Rocket_Simulation/Goanna_Rocket/Point Mass with Air Resistance Dynamics /Cd Estimator1/Rocket Specific Cd Estimator ==
  data: SA input; Cd output; V input; rho input
function Cd = fcn(SA,V,rho)
u1 =  43.32270126;  % Total rocket SA.
u2 = -0.000687709; % Velocity
u3 = 0.531869262; % Air density
intercept = -0.447146101;
Cd = (SA*u1)+ (V*u2)+ (rho*u3) + (intercept) ;
end

== matlab function Rocket_Simulation/MATLAB Function1 ==
  data: input input; output output
function output = fcn(input)
    persistent max_value; % This stores the maximum value across function calls
    persistent done; % This flag indicates if the maximum value has been finalized

    if isempty(max_value)
        max_value = input; % Initialize with the first input
    end

    if isempty(done)
        done = false; % Initialize the done flag
    end

    % output = 0;

    if ~done        
        if input >= max_value
            max_value = input; % Update the maximum value if the current input is larger
        else
            done = true; % Finalize the maximum value once input decreases
            % output = 1;
        end
    end

    output = max_value; % Output the maximum value
end

== matlab function Rocket_Simulation/Controller/Velocity Planner/MATLAB Function2 ==
  data: area input; Cd_preds output; rho input; velocity input
function Cd_preds = predict_drag_coefficients(area, rho, velocity)
    % Load model parameters from the .mat file
    params = load('model_params.mat');
    velocity = abs(velocity); % Ensure velocities are positive
    
    % Generate predictions for a grid of velocities
    force_preds = arrayfun(@(v) poly_predict(area, rho, v, params), velocity);
    
    % Check if any of the inputs are zero
    if area ~= 0 && rho ~= 0 && all(velocity ~= 0)
        % Calculate Cd for each velocity
        Cd_preds = arrayfun(@(f, v) f / (0.5 * rho * area * v^2), force_preds, velocity);
        
        % Ensure all Cd_preds are positive
        Cd_preds(Cd_preds <= 0) = 0.386598;
    else
        % Assign default value if any input is zero
        Cd_preds = 0.386598 * ones(size(velocity));
    end
end

function y_pred = poly_predict(area, rho, velocity, params)
    % Extract the parameters
    scaler_X_mean = params.scaler_X_mean;
    scaler_X_std = params.scaler_X_std;
    scaler_y_mean = params.scaler_y_mean;
    scaler_y_std = params.scaler_y_std;
    coefficients = params.coefficients;
    intercept = params.intercept;

    % Standardize input features (This is required because the GPR was trained this way)
    X = [(area - scaler_X_mean(1)) / scaler_X_std(1), ...
         (rho - scaler_X_mean(2)) / scaler_X_std(2), ...
         (velocity - scaler_X_mean(3)) / scaler_X_std(3)];

    % Compute polynomial features up to the desired degree
    degree = 3;
    X_poly = get_poly_features(X, degree);

    % Predict using the polynomial model
    y_scaled = sum(coefficients .* X_poly) + intercept;

    % Inverse standardization of the prediction
    y_pred = y_scaled * scaler_y_std + scaler_y_mean;
end

function X_poly = get_poly_features(X, degree)
    % Generate polynomial features up to the desired degree
    n = length(X);
    X_poly = 1;  % constant bias term

    for d = 1:degree
        combos = nchoosek(repmat(1:n, 1, d), d);
        combos = unique(sort(combos, 2), 'rows');
        for i = 1:size(combos, 1)
            term = prod(X(combos(i, :)));
            X_poly = [X_poly, term];
        end
    end
end

== matlab function Rocket_Simulation/Controller/Velocity Tracker/MATLAB Function2 ==
  data: x input; K output
function K = GainSchedulingPolynomialAlgorithm(x)
%#codegen
%k = Gain 
%X =  rocket velocity

% Define the coefficients
a = -1e-5;
b = 0.0037;
c = -0.3743;

% Compute the quadratic equation
K = a*x^2 + b*x + c;

== matlab function Rocket_Simulation/Controller/Velocity Planner/MATLAB Function4 ==
  data: area input; force_preds output; rho input; velocity input
function force_preds = predict_drag_coefficients(area, rho, velocity)
    area = abs(area);
    % Load model parameters from the .mat file
    params = load('force_pred.mat');
    velocity = abs(velocity); % Ensure velocities are positive

    if velocity >= 30
        % Generate predictions for a grid of velocities
        force_preds = arrayfun(@(v) poly_predict(area, rho, v, params), velocity);
    else
        force_preds = 0;
    end
   
    if force_preds < 0
        force_preds = 0.0;
    elseif isnan(force_preds)
        force_preds = 0.0;
    end

    if force_preds > 1000
        disp(force_preds)
        disp(area)
        disp(rho)
        disp(velocity)
    end
end

function y_pred = poly_predict(area, rho, velocity, params)
    % Extract the parameters
    scaler_X_mean = params.scaler_X_mean;
    scaler_X_std = params.scaler_X_std;
    scaler_y_mean = params.scaler_y_mean;
    scaler_y_std = params.scaler_y_std;
    coefficients = params.coefficients;
    intercept = params.intercept;

    % Standardize input features (This is required because the GPR was trained this way)
    X = [(area - scaler_X_mean(1)) / scaler_X_std(1), ...
         (rho - scaler_X_mean(2)) / scaler_X_std(2), ...
         (velocity - scaler_X_mean(3)) / scaler_X_std(3)];

    % Compute polynomial features up to the desired degree
    degree = 3;
    X_poly = get_poly_features(X, degree);

    % Predict using the polynomial model
    y_scaled = sum(coefficients .* X_poly) + intercept;

    % Inverse standardization of the prediction
    y_pred = y_scaled * scaler_y_std + scaler_y_mean;
end

function X_poly = get_poly_features(X, degree)
    % Generate polynomial features up to the desired degree
    n = length(X);
    X_poly = 1;  % constant bias term

    for d = 1:degree
        combos = nchoosek(repmat(1:n, 1, d), d);
        combos = unique(sort(combos, 2), 'rows');
        for i = 1:size(combos, 1)
            term = prod(X(combos(i, :)));
            X_poly = [X_poly, term];
        end
    end
end

== matlab function Rocket_Simulation/Controller/Velocity Planner/BT_Cd Estimator1/Rocket Specific Cd Estimator ==
  data: SA input; Cd output; V input; rho input
function Cd = fcn(SA,V,rho)
u1 =  43.32270126;  % Total rocket SA.
u2 = -0.000687709; % Velocity
u3 = 0.531869262; % Air density
intercept = -0.447146101;
Cd = (SA*u1)+ (V*u2)+ (rho*u3) + (intercept) ;
end

== matlab function Rocket_Simulation/target apogee changer ==
  data: initial_target input; input input; new_target_apogee output; delta_threshold input; time_threshold input; Ts input
function new_target_apogee = detectSteadyState(initial_target, input, delta_threshold, time_threshold, Ts)
    % Persistent variables to store previous value and time in steady state
    persistent prev_input time_in_steady_state done;

    if  isempty(done)
        done = false;
    end

    if isempty(prev_input)
        prev_input = input;
        time_in_steady_state = 0;
    end

    if ~done        
        % Calculate the difference between current and previous input
        delta = abs(input - prev_input);
        
        % Check if the difference is within the delta_threshold
        if delta < delta_threshold
            % Accumulate time in steady state
            time_in_steady_state = time_in_steady_state + Ts;
        else
            % Reset the time in steady state if condition is not met
            time_in_steady_state = 0;
        end
        
        % Update the previous input for the next iteration
        prev_input = input;
        
        % Initialize the new target apogee with the initial target value
        new_target_apogee = initial_target;
        
        % Check if the time in steady state exceeds the time_threshold
        if time_in_steady_state >= time_threshold
            % We are in steady state
            
            predicted_apogee = input;
    
            % Define the tolerance range (10% of the initial target)
            tolerance = 0.1 * initial_target;
            
            % Check if the predicted apogee is within 10% of the initial target
            if predicted_apogee < (initial_target)
                % If predicted apogee is more than 10% lower than the initial target,
                % set the new target apogee to the predicted apogee
                new_target_apogee = predicted_apogee * 0.9;
                prev_input = new_target_apogee;
                done = true;
            elseif predicted_apogee > (initial_target + tolerance)
                % If predicted apogee is more than 10% higher than the initial target,
                % set the new target apogee to 90% of the predicted apogee
                new_target_apogee = predicted_apogee * 0.9;
                prev_input = new_target_apogee;
                done = true;
            end
        end
    else
        new_target_apogee = prev_input;
    end

end
